simulink model "simulation"  (R2025b)
settings: Solver=VariableStepAuto  StartTime=0.0  StopTime=1e-5  RelTol=1e-3
libraries: commchan3 x1, commdigbbndapm x1, commfilt2 x1, commrandsrc3 x1
settings Model: Creator=Panos  LastModifiedBy=Panos

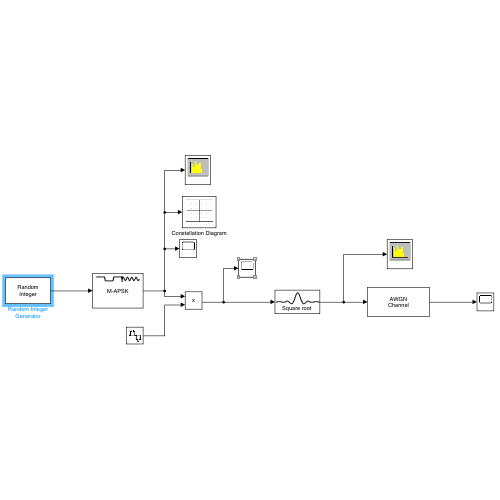
[thumbnail: Simulink's stored preview of the top-level diagram]
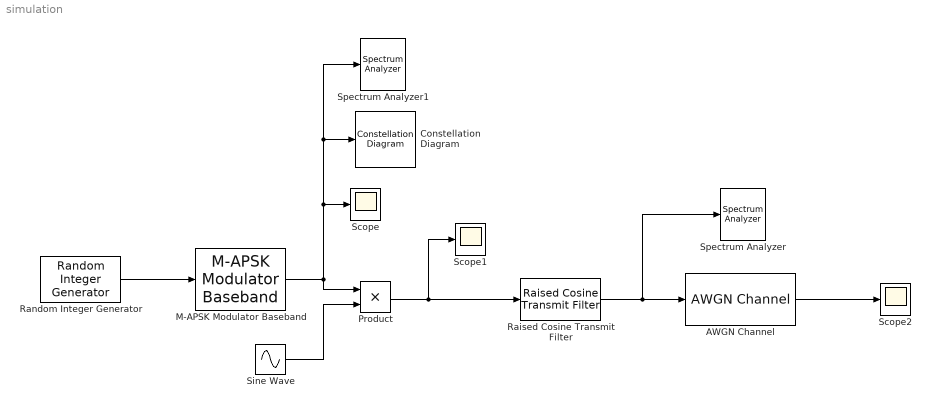
== system simulation ==
  AWGN Channel : commchan3/AWGN Channel  LegacyMode=off  NoiseMethod="Signal to noise ratio  (SNR)"  noiseMode="Signal to noise ratio  (SNR)"  EbNo=10  EsNo=10  SNR=30  BitsPerSymbol=1  SignalPower=1  SpecifySymbolPeriod=off  SamplesPerSymbol=1  SymbolPeriod=1  VarianceSource=Parameter  Variance=1  RandomStream=Global stream  Seed=67  SimulateUsing=Code generation
  Constellation Diagram : ConstellationDiagram  WindowPosition=[1.000000,49.000000,2048.000000,1081.000000,]  ScopeFrameLocation=window  SymbolsToDisplaySource=Property  SymbolsToDisplay=1000  ShowLegend=on
  M-APSK Modulator Baseband : commdigbbndapm/M-APSK Modulator Baseband  ConstPointsCirclewise=[32, 32, 32, 32, 32, 32, 32, 32]  Radii=[1, 1.791, 2.405, 2.980, 3.569, 4.235, 5.078, 6.536]  PhaseOffset=mod([1*pi/32, 3*pi/32, 5*pi/32, 7*pi/32, 9*pi/32, 11*pi/32, 13*pi/32, 15*pi/32], 2*pi./[32, 32, 32, 32, 32, 32, 32, 32])  SymbolMapping=Auto  CustomSymbolMapping=[ 0, 4, 12, 8, 1, 3, 2, 6, 7, 5, 13, 15, 14, 10, 11, 9 ]  InputType=Integer  OutputDataType=double  SimulateUsing=Code generation
  Product : Product
  Raised Cosine Transmit Filter : commfilt2/Raised Cosine Transmit Filter  filtType=Square root  R=0.2  filtSpan=16  N=8  filterGain=1  InputProcessing=Columns as channels (frame based)  RateOptions=Allow multirate processing  framing=Mute  checkCoeff=off  variableName=rcTxFilt  checkGain=Normalized  sampMode=Mute  saveAsFlag=0  currentFiltSpan=10  D=(10)/2  launchFVT=on  roundingMode=Floor  overflowMode=off  coeffDataTypeStr=Inherit: Same word length as input  coeffMin=[]  coeffMax=[]  coeffLastDataTypeStr=Inherit: Same word length as input  outputDataTypeStr=Inherit: Same as accumulator  outputMin=[]  outputMax=[]  outputLastDataTypeStr=Inherit: Same as accumulator
  Random Integer Generator : commrandsrc3/Random Integer Generator  SetSize=256  SeedSource=Auto  Seed=0  SampleTime=8e-9  SamplesPerFrame=1  OutputDataType=double  SimulateUsing=Interpreted execution
  Scope : Scope
      settings: ActiveDisplayYMinimum=-8.1306592169118481  ActiveDisplayYMaximum=8.1306592169118481
  Scope1 : Scope
      settings: ActiveDisplayYMinimum=-7.1137650990564758  ActiveDisplayYMaximum=9.1462694130779862
  Scope2 : Scope
      settings: ActiveDisplayYMinimum=-4.7857239331205506  ActiveDisplayYMaximum=4.6244722605487549  DataLoggingVariableName=ScopeData2
  Sine Wave : Sin  Frequency=2*pi*11.2e9  SampleTime=1e-11
  Spectrum Analyzer : SpectrumAnalyzer  WindowPosition=[1.000000,49.000000,2048.000000,1081.000000,]  ScopeFrameLocation=window  PlotAsTwoSidedSpectrum=off  WindowInvariantSamplesPerUpdate=on  Span=100000000000  StartFrequency=-50000000000  StopFrequency=50000000000  YLimits=[-146.4104 33.3969]  ShowLegend=on
  Spectrum Analyzer1 : SpectrumAnalyzer  WindowPosition=[1.000000,49.000000,2048.000000,1081.000000,]  ScopeFrameLocation=window  SampleRateSource=Property  SampleRate=4000e6  WindowInvariantSamplesPerUpdate=on  Span=100000000000  StartFrequency=-50000000000  StopFrequency=50000000000  YLimits=[-39.5185 13.5479]  ShowLegend=on
  wires:
  Random Integer Generator/1 -> M-APSK Modulator Baseband/1
  Sine Wave/1 -> Product/2
  M-APSK Modulator Baseband/1 -> Product/1, Spectrum Analyzer1/1, Constellation Diagram/1, Scope/1
  Product/1 -> Raised Cosine Transmit Filter/1, Scope1/1
  AWGN Channel/1 -> Scope2/1
  Raised Cosine Transmit Filter/1 -> Spectrum Analyzer/1, AWGN Channel/1
